simulink model "Angelo_Tulbure_Project_Simulink"  (R2021b)
settings: Solver=VariableStepAuto  StartTime=0.0  StopTime=1  RelTol=1e-3
values from neighbouring files (symbols this model uses):
  denomR = RR.Denominator    [Angelo_Tulbure_Project_MATLAB.m]
  GG = tf(sys)    [Angelo_Tulbure_Project_MATLAB.m]
  GG_numeratore = GG.Numerator    [Angelo_Tulbure_Project_MATLAB.m]
  numR = RR.Numerator    [Angelo_Tulbure_Project_MATLAB.m]
  ue = cfe    (= 0)    [Angelo_Tulbure_Project_MATLAB.m]
  x1e = nse    (= 50)    [Angelo_Tulbure_Project_MATLAB.m]
  x2e = nre    (= 50)    [Angelo_Tulbure_Project_MATLAB.m]
settings Model: Creator=angelo  LastModifiedBy=angelo

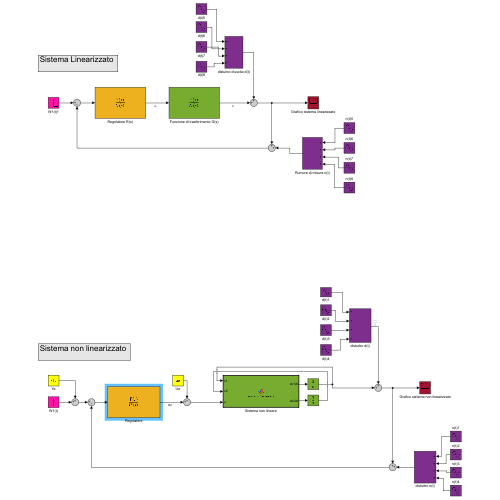
[thumbnail: Simulink's stored preview of the top-level diagram]
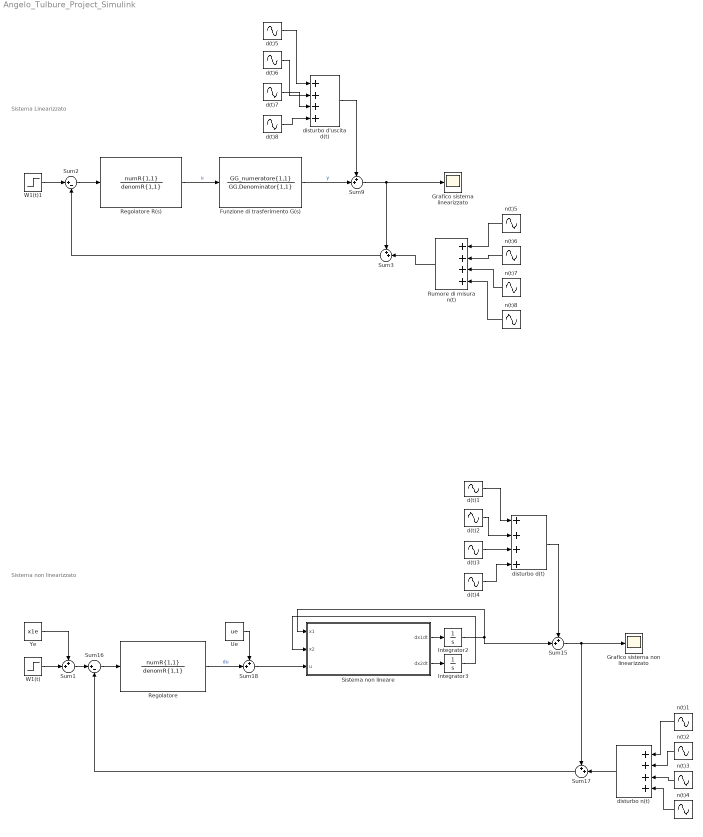
== system Angelo_Tulbure_Project_Simulink ==
  note: Sistema Linearizzato
  note: Sistema non linearizzato
  Funzione di trasferimento G(s) : TransferFcn  Numerator=GG_numeratore{1,1}  Denominator=GG.Denominator{1,1}
  Grafico sistema linearizzato : Scope
  Grafico sistema non linearizzato : Scope
  Integrator2 : Integrator  InitialCondition=x1e
  Integrator3 : Integrator  InitialCondition=x2e
  Regolatore : TransferFcn  Numerator=numR{1,1}  Denominator=denomR{1,1}
  Regolatore R(s) : TransferFcn  Numerator=numR{1,1}  Denominator=denomR{1,1}
  Rumore di misura n(t) : Sum  Inputs=++++
  Sistema non lineare : MATLAB Function  TreatAsAtomicUnit=on
  Sum{1,3,9,15,17..18} (6 alike) : Sum  Inputs=++|
  Sum16 : Sum  Inputs=|+-
  Sum2 : Sum  Inputs=|+-
  Ue : Constant  Value=ue
  W1(t) : Step  Time=0  After=-2  SampleTime=0
  W1(t)1 : Step  Time=0  After=-2  SampleTime=0
  Ye : Constant  Value=x1e
  d(t)1 : Sin  Amplitude=0.3  Frequency=(0.01875)*1  SampleTime=0
  d(t)2 : Sin  Amplitude=0.3  Frequency=(0.01875)*2  SampleTime=0
  d(t)3 : Sin  Amplitude=0.3  Frequency=(0.01875)*3  SampleTime=0
  d(t)4 : Sin  Amplitude=0.3  Frequency=(0.01875)*4  SampleTime=0
  d(t)5 : Sin  Amplitude=0.3  Frequency=(0.01875)*1  SampleTime=0
  d(t)6 : Sin  Amplitude=0.3  Frequency=(0.01875)*2  SampleTime=0
  d(t)7 : Sin  Amplitude=0.3  Frequency=(0.01875)*3  SampleTime=0
  d(t)8 : Sin  Amplitude=0.3  Frequency=(0.01875)*4  SampleTime=0
  disturbo d'uscita d(t) : Sum  Inputs=++++
  disturbo d(t) : Sum  Inputs=++++
  disturbo n(t) : Sum  Inputs=++++
  n(t)1 : Sin  Amplitude=0.2  Frequency=(1.5*10^4)*1  SampleTime=0
  n(t)2 : Sin  Amplitude=0.2  Frequency=(1.5*10^4)*2  SampleTime=0
  n(t)3 : Sin  Amplitude=0.2  Frequency=(1.5*10^4)*3  SampleTime=0
  n(t)4 : Sin  Amplitude=0.2  Frequency=(1.5*10^4)*4  SampleTime=0
  n(t)5 : Sin  Amplitude=0.2  Frequency=(1.5*10^4)*1  SampleTime=0
  n(t)6 : Sin  Amplitude=0.2  Frequency=(1.5*10^4)*2  SampleTime=0
  n(t)7 : Sin  Amplitude=0.2  Frequency=(1.5*10^4)*3  SampleTime=0
  n(t)8 : Sin  Amplitude=0.2  Frequency=(1.5*10^4)*4  SampleTime=0
  wires:
  Sistema non lineare/1(dx1dt) -> Integrator2/1
  n(t)1/1 -> disturbo n(t)/1
  Sum16/1 -> Regolatore/1
  Sum15/1 -> Grafico sistema non linearizzato/1, Sum17/1
  Sum18/1 -> Sistema non lineare/3(u)
  Integrator2/1 -> Sistema non lineare/1(x1), Sum15/2
  Sum2/1 -> Regolatore R(s)/1
  n(t)3/1 -> disturbo n(t)/3
  n(t)6/1 -> Rumore di misura n(t)/2
  Regolatore/1 -> Sum18/2  "du"
  disturbo n(t)/1 -> Sum17/2
  Regolatore R(s)/1 -> Funzione di trasferimento G(s)/1  "u"
  n(t)2/1 -> disturbo n(t)/2
  d(t)4/1 -> disturbo d(t)/4
  disturbo d(t)/1 -> Sum15/1
  d(t)1/1 -> disturbo d(t)/1
  n(t)4/1 -> disturbo n(t)/4
  d(t)2/1 -> disturbo d(t)/2
  Sum3/1 -> Sum2/2
  Sum9/1 -> Grafico sistema linearizzato/1, Sum3/1
  n(t)5/1 -> Rumore di misura n(t)/1
  Integrator3/1 -> Sistema non lineare/2(x2)
  Sistema non lineare/2(dx2dt) -> Integrator3/1
  n(t)7/1 -> Rumore di misura n(t)/3
  Ue/1 -> Sum18/1
  n(t)8/1 -> Rumore di misura n(t)/4
  disturbo d'uscita d(t)/1 -> Sum9/1
  d(t)6/1 -> disturbo d'uscita d(t)/2
  Funzione di trasferimento G(s)/1 -> Sum9/2  "y"
  d(t)7/1 -> disturbo d'uscita d(t)/3
  Rumore di misura n(t)/1 -> Sum3/2
  d(t)8/1 -> disturbo d'uscita d(t)/4
  d(t)5/1 -> disturbo d'uscita d(t)/1
  W1(t)1/1 -> Sum2/1
  d(t)3/1 -> disturbo d(t)/3
  Ye/1 -> Sum1/1
  W1(t)/1 -> Sum1/2
  Sum1/1 -> Sum16/1
  Sum17/1 -> Sum16/2

== matlab function Angelo_Tulbure_Project_Simulink/Sistema non lineare ==
  data: x1 input; x2 input; u input; dx1dt output; dx2dt output
function [dx1dt, dx2dt] = systemDynamics(x1, x2, u)

rs = 1.2;       %tasso di riproduzione cellule suscettibili
rr = 1.1;       %tasso di riproduzione cellule resistenti
k = 100;        %numero massimo di cellule 
gamma = 0.1;    %cambio da resistenti a suscettibili
beta = 0.1;     %cambio da suscettibili a resistenti
alpha = 0.1;    %cambio da suscettibili a resistenti dopo trattamento farmacologico
ms = 0.8;       %mortalità cellule suscettibili
mr = 0.1;       %mortalità cellule resistenti


dx1dt = rs*(1-(x1+x2)/k)*x1-ms*u*x1-beta*x1+gamma*x2-alpha*u*x1;
dx2dt = rr*(1-(x1+x2)/k)*x2-mr*u*x2+beta*x1-gamma*x2+alpha*u*x1;
